simulink subsystem "Sonars"  (R2023b)
settings: Solver=VariableStepAuto  StartTime=0.0  StopTime=10.0  RelTol=1e-3
libraries: arduinolib x2
settings Model: Creator=Carlos  LastModifiedBy=adria

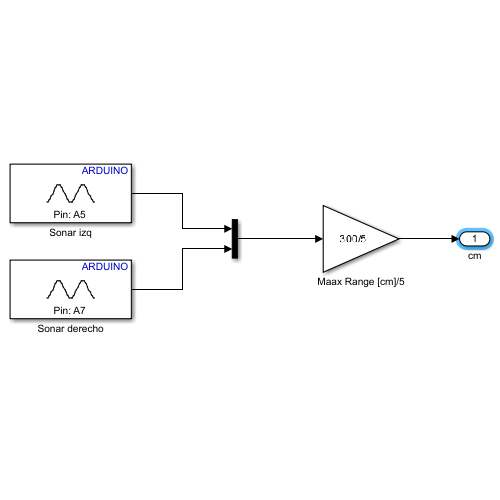
[thumbnail: Simulink's stored preview of the top-level diagram]
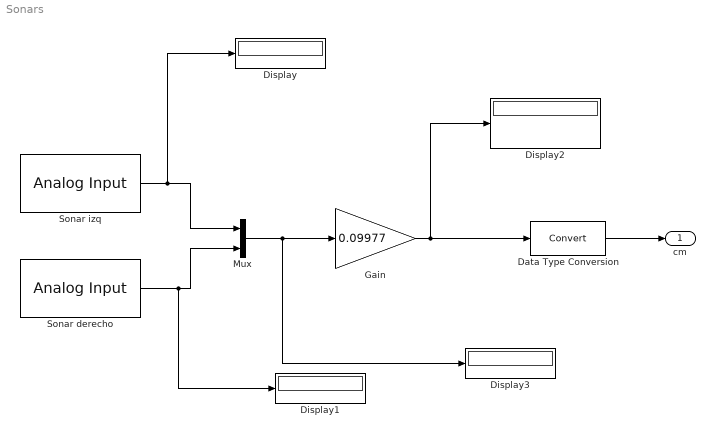
== system Sonars ==
  Data Type Conversion : DataTypeConversion  SaturateOnIntegerOverflow=off  RndMeth=Floor
  Display{,1..3} (4 alike) : Display
  Gain : Gain  Gain=0.09977
  Mux : Mux  Inputs=2
  Sonar derecho : arduinolib/Analog Input  pinNumber=0  ReadResultsOnly=off  ConversionTriggerSource=Software  ExternalTriggerType=uint32( 0 )  OutputDataType=uint16  EnableConversionCompleteNotify=off  EnableOuputStatus=off  SampleTime=.1  blockPlatform=arduino
  Sonar izq : arduinolib/Analog Input  pinNumber=1  ReadResultsOnly=off  ConversionTriggerSource=Software  ExternalTriggerType=uint32( 0 )  OutputDataType=uint16  EnableConversionCompleteNotify=off  EnableOuputStatus=off  SampleTime=.1  blockPlatform=arduino
  cm : Outport  OutDataTypeStr=int16
  wires:
  Mux/1 -> Gain/1, Display3/1
  Sonar izq/1 -> Mux/1, Display/1
  Sonar derecho/1 -> Mux/2, Display1/1
  Gain/1 -> Display2/1, Data Type Conversion/1
  Data Type Conversion/1 -> cm/1
